simulink model "Autopilot_harness"  (Simulink 8.0)
settings: Solver=ode23  StartTime=0.0  StopTime=25  MaxStep=1/40  RelTol=1e-2  AbsTol=1e-3
model workspace (MAT data in the model file):
  tmp20121902TempDataBlockParam15378051 = 1
  tmp20121902TempDataBlockParam16564336 = 1
  tmp20121902TempDataBlockParam11960188 = 1
  beaver_init_roll = 0
  tmp2399823TempDataBlockParam8793363 = 1
  tmp2399823TempDataBlockParam27430435 = 11
  tmp2399823TempDataBlockParam30328219 : num (value not decoded)
PreLoadFcn:
  | Plant_data
values from neighbouring files (symbols this model uses):
  beaver_init_roll = 0    [Plant_data.m]
undefined symbols (not defined in the file or in its folder): sigbuilder_block
libraries: simulink x4, aerolibconvert2 x1, Plant x1
Description:
  | Fly the DeHavilland Beaver
  | 
  | This demonstration uses a pilot's joystick to allow you to fly the DeHavilland
  | Beaver modeled with Simulnk, and Aerospace Blockset.  This model has been
  | color coded to aid in locating Aerospace Blockset blocks. The red blocks are
  | Aerospace Blockset blocks, the orange blocks are subsystems containing
  | additional Aerospace Blockset blocks and the white blocks are Simulink blocks.
  | 
  | The DeHavilland Beaver model includes the airframe dynamics, including
  | aerodynamics. Effects of the environment are also modeled, such as wind profiles
  | for the landing phase. Visualization for this model is done via an interface to
  | FlightGear, a open source flight simulator package.
  | 
  | The DeHavilland Beaver was first flown in 1947. Today it is still prized by pilots
  | for its reliability and versatility. The DeHavilland Beaver can be operated on wheels,
  | skis or float landing gear.
  | 
  | Speed Max       110 kts
  | Altitude Max 10,000 ft
  | Range Max       400 nm
  | Load                     6 passengers
  | Crew                     1 member
  | 
  | For more information on the FlightGear interface, see the documentation.
settings Model: Creator=The MathWorks Inc.  LastModifiedBy=ssauvage  CovMetricSettings=dcmtrwe  CovHTMLOptions=-aTS=1 -bRG=1 -bTC=1 -hTR=0 -nFC=0 -scm=1 -bcm=1 -xEv=0  CovSaveSingleToWorkspaceVar=off  CovCumulativeReport=on  CovModelRefEnable=off  ExtModeTrigMode=oneshot  ExtModeArmWhenConnect=off  ExtModeAutoUpdateStatusClock=off
settings DataIOCC: LimitDataPoints=off  SignalLoggingSaveFormat=ModelDataLogs  SaveOutput=off  SaveTime=off  SignalLoggingName=tmp2399823SignalLoggingName
settings OptimizationCC: BlockReduction=off  ConditionallyExecuteInputs=off  InlineParams=on  UseIntDivNetSlope=on  InlineInvariantSignals=on  InitFltsAndDblsToZero=on  EfficientFloat2IntCast=on  OptimizeModelRefInitCode=on
settings DebuggingCC: SignalInfNanChecking=error  ReadBeforeWriteMsg=EnableAllAsError  WriteAfterWriteMsg=EnableAllAsError  WriteAfterReadMsg=EnableAllAsError  AlgebraicLoopMsg=error  ArtificialAlgebraicLoopMsg=error  SaveWithParameterizedLinksMsg=none  CheckExecutionContextPreStartOutputMsg=on  CheckExecutionContextRuntimeOutputMsg=on  BlockPriorityViolationMsg=error  MaxConsecutiveZCsMsg=warning  InheritedTsInSrcMsg=error  DiscreteInheritContinuousMsg=error  SigSpecEnsureSampleTimeMsg=error  CheckMatrixSingularityMsg=error  IntegerOverflowMsg=error  ParameterUnderflowMsg=error  ParameterPrecisionLossMsg=error  UnnecessaryDatatypeConvMsg=warning  VectorMatrixConversionMsg=warning  SignalLabelMismatchMsg=warning  UnconnectedInputMsg=error  UnconnectedOutputMsg=error  UnconnectedLineMsg=error  SFcnCompatibilityMsg=warning  BusObjectLabelMismatch=error  RootOutportRequireBusObject=error  AssertControl=DisableAll  ModelReferenceIOMsg=error  ModelReferenceIOMismatchMessage=error  UnknownTsInhSupMsg=error  ModelReferenceDataLoggingMessage=error
settings HardwareCC: ProdIntDivRoundTo=Zero  ProdEndianess=LittleEndian  ProdHWDeviceType=Generic->Custom  TargetHWDeviceType=32-bit Generic
settings ModelReferenceCC: CheckModelReferenceTargetMessage=none
settings RTWCC: SystemTargetFile=ert.tlc  TemplateMakefile=ert_default_tmf  Description=Real-Time Workshop Embedded Coder (no auto configuration)  RTWVerbose=off  ProcessScript=ert_make_rtw_hook  IncludeERTFirstTime=on
settings CodeAppCC: ForceParamTrailComments=on  IgnoreCustomStorageClasses=off  MangleLength=4  ReqsInCode=on
settings ERTTargetCC: TargetFcnLib=ansi_tfl_tmw.mat  CodeReplacementLibrary=ANSI_C  MultiwordLength=2048  GenerateSampleERTMain=on  IncludeMdlTerminateFcn=off  SuppressErrorStatus=on  SupportAbsoluteTime=off  SupportNonFinite=off  SupportComplex=off  InlinedParameterPlacement=NonHierarchical  ERTCustomFileTemplate=example_file_process.tlc  ConvertIfToSwitch=off  SuppressUnreachableDefaultCases=off

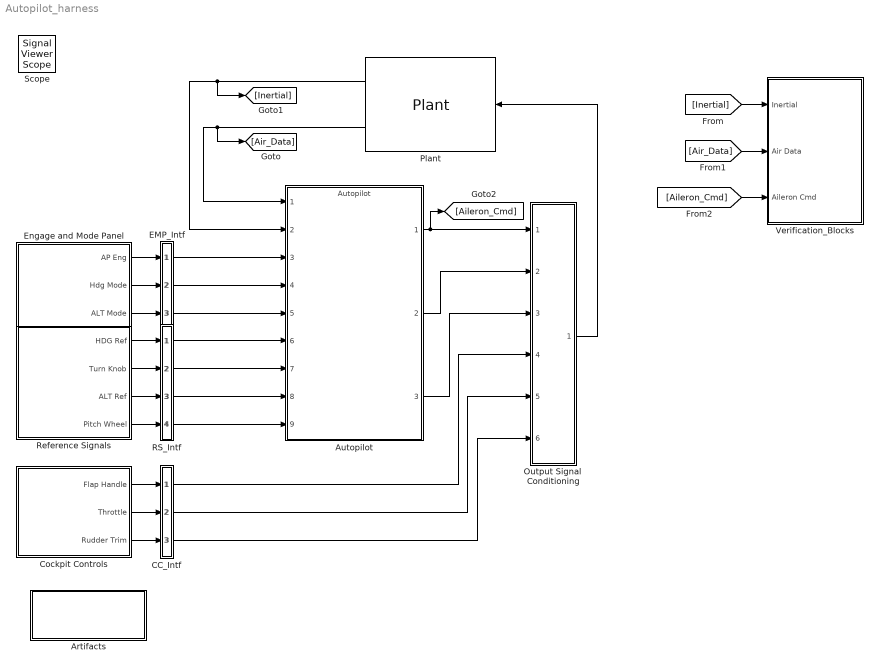
== system Autopilot_harness ==
  Artifacts : Subsystem
      mask Display: disp('View\nDO-178B Artifacts\n(double-click)');
  Autopilot : ModelReference  ModelNameDialog=Autopilot  SimulationMode=Normal  ModelReferenceVersion=1.155  CopyOfModelName=Autopilot  DefaultDataLogging=off
  CC_Intf : Subsystem
  Cockpit Controls : Subsystem  Tag=STV Subsys  LoadFcn=sigbuilder_block('load');  StartFcn=sigbuilder_block('start');  StopFcn=sigbuilder_block('stop');  ClipboardFcn=sigbuilder_block('clipboard');  mask(Sigbuilder block){}
      mask help: Sigbuilder GUI
      mask init:
      | if ~strcmp(get_param(bdroot(gcbh),'SimulationStatus'),'stopped') tuvar = sigbuilder_block('maskInit'); end
      settings: CopyFcn=sigbuilder_block('copy');  DeleteFcn=sigbuilder_block('delete');  ModelCloseFcn=sigbuilder_block('modelClose');  PreSaveFcn=sigbuilder_block('preSave');  PauseFcn=sigbuilder_block('pause')  ContinueFcn=sigbuilder_block('continue')  NameChangeFcn=sigbuilder_block('namechange');  OpenFcn=sigbuilder_block('open',[144.75 92.25 575.25 393 ]);  CloseFcn=sigbuilder_block('close');
      mask Display: plot(0,0,100,100,[10,10,40,40,10],[80,20,20,80,80],[40,10],[50,50], [40,27,10],[65,72,56],[40,25,25,10],[28,28,43,43]);
  EMP_Intf : Subsystem
  Engage and Mode Panel : Subsystem  Tag=STV Subsys  RequirementInfo={'other' 'do178b_autopilot_requirements.doc' '@1.2. Roll Hold Mode' 'true' '1.1. Roll Autopilot Engage Control' '' ; 'other' 'do178b_autopilot_requirements.doc' '1.2. Roll Hold Mode' 'true' '1.2. Roll Hold Mode' '' ; 'other' 'do178b_autopilot_requirements.doc' '1.1. Roll Autopilot Engage Control' 'true' '1.1. Roll Autopilot Engage Control' '' ; 'other' 'do178b_autopilot_requirements.doc' '1.8. Heading Hold Mode' 'true' '1.8. Heading Hold Mode' '' } %GIDa_8e9e9d99_d836_4084_a908_4b15c0f24bcd  LoadFcn=sigbuilder_block('load');  StartFcn=sigbuilder_block('start');  StopFcn=sigbuilder_block('stop');  ClipboardFcn=sigbuilder_block('clipboard');  mask(Sigbuilder block){}
      mask help: Sigbuilder GUI
      mask init:
      | if ~strcmp(get_param(bdroot(gcbh),'SimulationStatus'),'stopped') tuvar = sigbuilder_block('maskInit'); end
      settings: CopyFcn=sigbuilder_block('copy');  DeleteFcn=sigbuilder_block('delete');  ModelCloseFcn=sigbuilder_block('modelClose');  PreSaveFcn=sigbuilder_block('preSave');  PauseFcn=sigbuilder_block('pause')  ContinueFcn=sigbuilder_block('continue')  NameChangeFcn=sigbuilder_block('namechange');  OpenFcn=sigbuilder_block('open',[118.5 66 745.5 487.5 ]);  CloseFcn=sigbuilder_block('close');
      mask Display: plot(0,0,100,100,[10,10,40,40,10],[80,20,20,80,80],[40,10],[50,50], [40,27,10],[65,72,56],[40,25,25,10],[28,28,43,43]);
  Output Signal  Conditioning : Subsystem
  Plant : Plant/Plant  SystemSampleTime=-1
  RS_Intf : Subsystem
  Reference Signals : Subsystem  Tag=STV Subsys  RequirementInfo={'other' 'do178b_autopilot_requirements.doc' '1.3. Roll Hold Reference' 'true' '1.3. Roll Hold Reference' '' ; 'other' 'do178b_autopilot_requirements.doc' '1.9. Heading Hold Reference' 'true' '1.9. Heading Hold Reference' '' ; 'other' 'do178b_autopilot_requirements.doc' '1.3. Roll Hold Reference' 'true' '1.3. Roll Hold Reference' '' ; 'other' 'do178b_autopilot_requirements.doc' '1.3. Roll Hold Reference' 'true' '1.3. Roll Hold Reference' '' ; 'other' 'do178b_autopilot_requirements.doc' '1.3. Roll Hold Reference' 'true' '1.3. Roll Hold Reference' '' ; 'other' 'do178b_autopilot_requirements.doc' '1.3. Roll Hold Reference' 'true' '1.3. Roll Hold Reference' '' ; 'other' 'do178b_autopilot_requirements.doc' '1.3. Roll Hold Reference' 'true' '1.3. Roll Hold Reference' '' ; 'other' 'do178b_autopilot_requirements.doc' '1.3. Roll Hold Reference' 'true' '1.3. Roll Hold Reference' '' ; 'other' 'do178b_autopilot_requirements.doc' '1.4. Roll Performance' 'true' '1.4. Roll Performance' '' ; 'other' 'do178b_autopilot_requirements.doc' '1.4. Roll Performance' 'true' '1.4. Roll Performance' '' ; 'other' 'do178b_autopilot_requirements.doc' '1.4. Roll Performance' 'true' '1.4. Roll Performance' '' ; 'other' 'do178b_autopilot_requirements.doc' '1.5. Roll Rate Limit' 'true' '1.5. Roll Rate Limit' '' ; 'other' 'do178b_autopilot_requirements.doc' '1.6. Roll Angle Limit' 'true' '1.6. Roll Angle Limit' '' ; 'other' 'do178b_autopilot_requirements.doc' '1.4. Roll Performance' 'true' '1.4. Roll Performance' '' ; 'other' 'do178b_autopilot_requirements.doc' '1.5. Roll Rate Limit' 'true' '1.5. Roll Rate Limit' '' ; 'other' 'do178b_autopilot_requirements.doc' '1.6. Roll Angle Limit' 'true' '1.6. Roll Angle Limit' '' } %GIDa_9d9b9e1a_9cda_4488_bbc7_0b4cdaadb6f4  LoadFcn=sigbuilder_block('load');  StartFcn=sigbuilder_block('start');  StopFcn=sigbuilder_block('stop');  ClipboardFcn=sigbuilder_block('clipboard');  mask(Sigbuilder block){}
      mask help: Sigbuilder GUI
      mask init:
      | if ~strcmp(get_param(bdroot(gcbh),'SimulationStatus'),'stopped') tuvar = sigbuilder_block('maskInit'); end
      settings: CopyFcn=sigbuilder_block('copy');  DeleteFcn=sigbuilder_block('delete');  ModelCloseFcn=sigbuilder_block('modelClose');  PreSaveFcn=sigbuilder_block('preSave');  PauseFcn=sigbuilder_block('pause')  ContinueFcn=sigbuilder_block('continue')  NameChangeFcn=sigbuilder_block('namechange');  OpenFcn=sigbuilder_block('open',[124.5 -29.25 745.5 487.5 ]);  CloseFcn=sigbuilder_block('close');
      mask Display: plot(0,0,100,100,[10,10,40,40,10],[80,20,20,80,80],[40,10],[50,50], [40,27,10],[65,72,56],[40,25,25,10],[28,28,43,43]);
  Verification_Blocks : Subsystem
  Scope : SignalViewerScope  IOType=viewer  ZoomMode=yonly  RefreshTime=0.035000
  wires:
  Output Signal  Conditioning/1(Controls) -> Plant/1
  Autopilot/1 -> Output Signal  Conditioning/1(Aileron), [Aileron_Cmd]
  Plant/2 -> [Air_Data], Autopilot/1
  Plant/1 -> [Inertial], Autopilot/2
  Autopilot/2 -> Output Signal  Conditioning/2(Elevator)
  Autopilot/3 -> Output Signal  Conditioning/3(Rudder)
  Cockpit Controls/1(Flap Handle) -> CC_Intf/1(Flap Handle)
  Cockpit Controls/2(Throttle) -> CC_Intf/2("Throttle ")
  Engage and Mode Panel/1(AP Eng) -> EMP_Intf/1(AP Eng)
  Engage and Mode Panel/2(Hdg Mode) -> EMP_Intf/2(Hdg Mode)
  Engage and Mode Panel/3(ALT Mode) -> EMP_Intf/3(ALT Mode)
  Reference Signals/1(HDG Ref) -> RS_Intf/1(HDG Ref)
  Reference Signals/2(Turn Knob) -> RS_Intf/2(Turn Knob)
  Reference Signals/3(ALT Ref) -> RS_Intf/3(ALT Ref)
  Reference Signals/4(Pitch Wheel) -> RS_Intf/4(Pitch Wheel)
  EMP_Intf/1(AP_Eng) -> Autopilot/3
  EMP_Intf/2(Hdg_Mode) -> Autopilot/4
  EMP_Intf/3(ALT_Mode) -> Autopilot/5
  RS_Intf/1(HDG_Ref) -> Autopilot/6
  RS_Intf/2(Turn_Knob) -> Autopilot/7
  RS_Intf/3(ALT_Ref) -> Autopilot/8
  RS_Intf/4(Pitch_Wheel) -> Autopilot/9
  Cockpit Controls/3(Rudder Trim) -> CC_Intf/3(Rudder Trim)
  CC_Intf/1(Flap_Handle) -> Output Signal  Conditioning/4(Flap)
  CC_Intf/2(Throttle) -> Output Signal  Conditioning/5(Throttle)
  CC_Intf/3(Rudder_Trim) -> Output Signal  Conditioning/6(Rudder Trim)
  [Inertial] -> Verification_Blocks/1(Inertial)
  [Air_Data] -> Verification_Blocks/2(Air Data)
  [Aileron_Cmd] -> Verification_Blocks/3(Aileron Cmd)

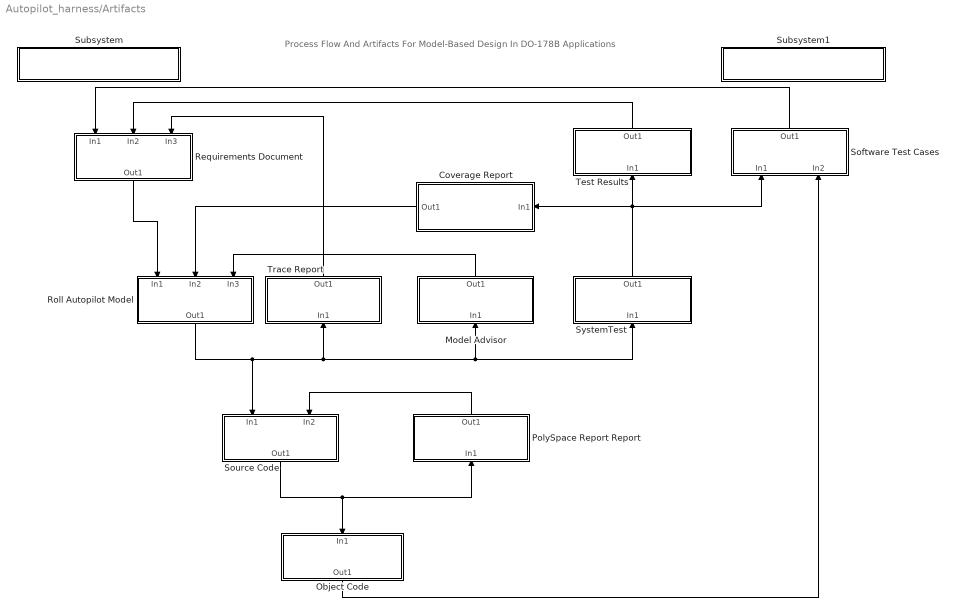
== system Autopilot_harness/Artifacts ==
  note: Process Flow And Artifacts For Model-Based Design In DO-178B Applications
  Coverage Report : Subsystem
      settings: OpenFcn=open('DO178B_Demo10203610.html');
      mask Display: disp('Open Model Coverage \nReport for Roll_AP \n (double-click)')
  Model Advisor : Subsystem
      settings: OpenFcn=|
      | open_system('roll_ap');
      | modeladvisor('roll_ap');
      mask Display: disp('Open Model Advisor \n for Roll_AP \n (double-click)')
  Object Code : Subsystem
      mask Display: disp('Compiled Object Code \n for Roll_AP')
  PolySpace Report Report : Subsystem
      settings: OpenFcn=winopen('results_roll_ap\misra_stats.csv');
      mask Display: disp('Polyspace Report \n for Roll_AP Code \n (double-click)')
  Requirements Document : Subsystem
      settings: OpenFcn=winopen('do178b_autopilot_requirements.doc');
      mask Display: disp('Open Requirements \n Document for Roll_AP \n (double-click)')
  Roll Autopilot Model : Subsystem
      settings: OpenFcn=open_system('roll_ap');
      mask Display: disp('Open Roll \n Autopilot Model \n (double-click)')
  Software Test Cases : Subsystem
      settings: OpenFcn=winopen('roll_ap_testcases(1).xls');
      mask Display: disp('Open Software Test \n Cases for Roll_AP \n (double-click)')
  Source Code : Subsystem
      settings: OpenFcn=open([pwd '\roll_ap_ert_rtw\html\roll_ap_codegen_rpt.html']);
      mask Display: disp('Open Code \n for Roll_AP \n (double-click)')
  Subsystem : Subsystem
      mask Display: disp('DO-178B Development Aritifacts');
  Subsystem1 : Subsystem
      mask Display: disp('DO-178B Verification Aritifacts');
  SystemTest : Subsystem
      settings: OpenFcn=systemtest('DO178B_Demo');
      mask Display: disp('Open SystemTest\n for DO178B_DHC2 \n (double-click)')
  Test Results : Subsystem
      settings: OpenFcn=|
      | %open('do178b_testreport.pdf');
      | open([pwd '\DO178B_Demo_report\DO178B_Demo_report.html']);
      mask Display: disp('Test Results Reports \n for DO178B_DHC2 \n (double-click)')
  Trace Report : Subsystem
      settings: OpenFcn=open('roll_ap_reqreport.html');
      mask Display: disp('Open Requirements \n Report for Roll_AP \n (double-click)')
  wires:
  PolySpace Report Report/1(Out1) -> Source Code/2(In2)
  Coverage Report/1(Out1) -> Roll Autopilot Model/2(In2)
  Object Code/1(Out1) -> Software Test Cases/2(In2)
  Software Test Cases/1(Out1) -> Requirements Document/1(In1)
  SystemTest/1(Out1) -> Software Test Cases/1(In1), Coverage Report/1(In1), Test Results/1(In1)
  Source Code/1(Out1) -> PolySpace Report Report/1(In1), Object Code/1(In1)
  Roll Autopilot Model/1(Out1) -> Source Code/1(In1), SystemTest/1(In1), Model Advisor/1(In1), Trace Report/1(In1)
  Test Results/1(Out1) -> Requirements Document/2(In2)
  Model Advisor/1(Out1) -> Roll Autopilot Model/3(In3)
  Trace Report/1(Out1) -> Requirements Document/3(In3)
  Requirements Document/1(Out1) -> Roll Autopilot Model/1(In1)

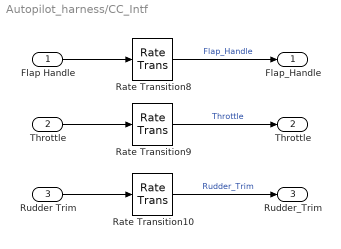
== system Autopilot_harness/CC_Intf ==
  Flap Handle : Inport
  "Throttle " : Inport  Port=2
  Rudder Trim : Inport  Port=3
  Rate Transition10 : RateTransition  OutPortSampleTime=1/40
  Rate Transition8 : RateTransition  OutPortSampleTime=1/40
  Rate Transition9 : RateTransition  OutPortSampleTime=1/40
  Flap_Handle : Outport
  Throttle : Outport  Port=2
  Rudder_Trim : Outport  Port=3
  wires:
  Flap Handle/1 -> Rate Transition8/1
  Rate Transition8/1 -> Flap_Handle/1  "Flap_Handle"
  "Throttle "/1 -> Rate Transition9/1
  Rate Transition9/1 -> Throttle/1  "Throttle"
  Rudder Trim/1 -> Rate Transition10/1
  Rate Transition10/1 -> Rudder_Trim/1  "Rudder_Trim"

== system Autopilot_harness/Cockpit Controls ==
  Demux : Demux  Tag=STV Demux  Outputs=3
  FromWs : FromWorkspace  Tag=STV FromWs  VariableName=tuvar  SampleTime=0  SigBuilderData=DataTag1  VnvData=DataTag2
      SigBuilderData=|
      | common.afterFinalStr = 'Extrapolate'
      | common.sampleTime = 0
      | dataSet.timeRange = [0 10]
      | dataSet.name = 'Steady State Flight'
      | sbobj.Groups.Name = 'Steady State Flight'
      | sbobj.Groups.Signals(1).Name = 'Flap Handle'
      | sbobj.Groups.Signals(1).XData = [0 10]
      | sbobj.Groups.Signals(1).YData = [0 0]
      | sbobj.Groups.Signals(2).Name = 'Throttle'
      | sbobj.Groups.Signals(2).XData = [0 10]
      | sbobj.Groups.Signals(2).YData = [0.625 0.625]
      | sbobj.Groups.Signals(3).Name = 'Rudder Trim'
      | sbobj.Groups.Signals(3).XData = [0 10]
      | sbobj.Groups.Signals(3).YData = [0 0]
  Flap Handle : Outport  Tag=STV Outport
  Throttle : Outport  Tag=STV Outport  Port=2
  Rudder Trim : Outport  Tag=STV Outport  Port=3
  wires:
  FromWs/1 -> Demux/1
  Demux/1 -> Flap Handle/1
  Demux/2 -> Throttle/1
  Demux/3 -> Rudder Trim/1

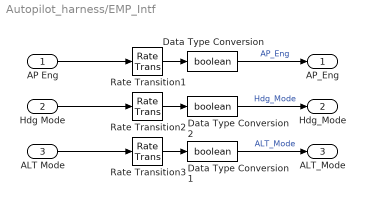
== system Autopilot_harness/EMP_Intf ==
  AP Eng : Inport
  Hdg Mode : Inport  Port=2
  ALT Mode : Inport  Port=3
  Data Type Conversion : DataTypeConversion  OutDataTypeStr=boolean
  Data Type Conversion1 : DataTypeConversion  OutDataTypeStr=boolean
  Data Type Conversion2 : DataTypeConversion  OutDataTypeStr=boolean
  Rate Transition1 : RateTransition  OutPortSampleTime=1/40
  Rate Transition2 : RateTransition  OutPortSampleTime=1/40
  Rate Transition3 : RateTransition  OutPortSampleTime=1/40
  AP_Eng : Outport
  Hdg_Mode : Outport  Port=2
  ALT_Mode : Outport  Port=3
  wires:
  AP Eng/1 -> Rate Transition1/1
  Data Type Conversion/1 -> AP_Eng/1  "AP_Eng"
  Hdg Mode/1 -> Rate Transition2/1
  Rate Transition2/1 -> Data Type Conversion2/1
  ALT Mode/1 -> Rate Transition3/1
  Rate Transition3/1 -> Data Type Conversion1/1
  Rate Transition1/1 -> Data Type Conversion/1
  Data Type Conversion2/1 -> Hdg_Mode/1  "Hdg_Mode"
  Data Type Conversion1/1 -> ALT_Mode/1  "ALT_Mode"

== system Autopilot_harness/Engage and Mode Panel ==
  Demux : Demux  Tag=STV Demux  Outputs=3
  FromWs : FromWorkspace  Tag=STV FromWs  VariableName=tuvar  SampleTime=0  SigBuilderData=DataTag3  VnvData=DataTag4
      SigBuilderData=|
      | common.afterFinalStr = 'Extrapolate'
      | common.sampleTime = 0
      | dataSet(1).timeRange = [0 25]
      | dataSet(1).name = 'Roll Hold Engage'
      | dataSet(2).timeRange = [0 25]
      | dataSet(2).name = 'Heading Hold Engage'
      | sbobj.Groups(1).Name = 'Roll Hold Engage'
      | sbobj.Groups(1).Signals(1).Name = 'AP Eng'
      | sbobj.Groups(1).Signals(1).XData = [0 0.1 0.1 25]
      | sbobj.Groups(1).Signals(1).YData = [0 0 1 1]
      | sbobj.Groups(1).Signals(2).Name = 'Hdg Mode'
      | sbobj.Groups(1).Signals(2).XData = [0 25]
      | sbobj.Groups(1).Signals(2).YData = [0 0]
      | sbobj.Groups(1).Signals(3).Name = 'ALT Mode'
      | sbobj.Groups(1).Signals(3).XData = [0 1 1 25]
      | sbobj.Groups(1).Signals(3).YData = [0 0 1 1]
      | sbobj.Groups(2).Name = 'Heading Hold Engage'
      | sbobj.Groups(2).Signals(1).Name = 'AP Eng'
      | sbobj.Groups(2).Signals(1).XData = [0 0.1 0.1 25]
      | sbobj.Groups(2).Signals(1).YData = [0 0 1 1]
      | sbobj.Groups(2).Signals(2).Name = 'Hdg Mode'
      | sbobj.Groups(2).Signals(2).XData = [0 1 1 25]
      | sbobj.Groups(2).Signals(2).YData = [0 0 1 1]
      | sbobj.Groups(2).Signals(3).Name = 'ALT Mode'
      | sbobj.Groups(2).Signals(3).XData = [0 1 1 25]
      | sbobj.Groups(2).Signals(3).YData = [0 0 1 1]
  AP Eng : Outport  Tag=STV Outport
  Hdg Mode : Outport  Tag=STV Outport  Port=2
  ALT Mode : Outport  Tag=STV Outport  Port=3
  wires:
  Demux/1 -> AP Eng/1
  FromWs/1 -> Demux/1
  Demux/2 -> Hdg Mode/1
  Demux/3 -> ALT Mode/1

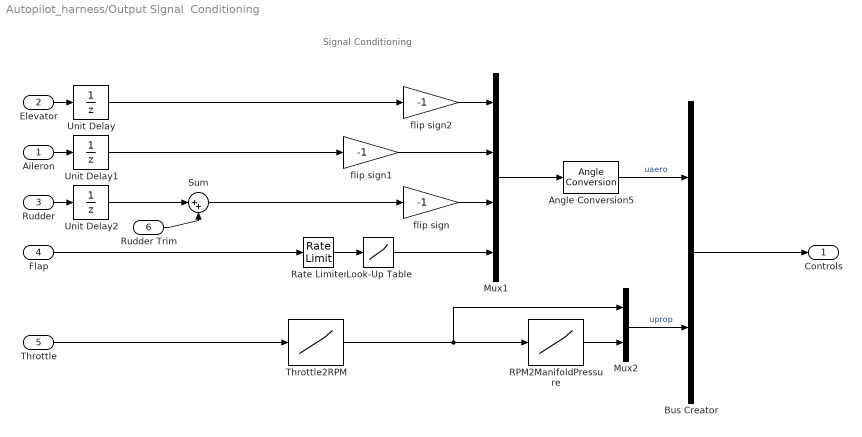
== system Autopilot_harness/Output Signal  Conditioning ==
  note: Signal Conditioning
  Aileron : Inport
  Elevator : Inport  Port=2
  Rudder : Inport  Port=3
  Flap : Inport  Port=4
  Throttle : Inport  Port=5
  Rudder Trim : Inport  Port=6
  Angle Conversion5 : aerolibconvert2/Angle Conversion  IU=deg  OU=rad
  Bus Creator : BusCreator  Inputs=2
  Look-Up Table : Lookup  InputValues=[0:3]  Table=[0 4 10 20]  SaturateOnIntegerOverflow=on
  Mux1 : Mux
  Mux2 : Mux  Inputs=2
  RPM2ManifoldPressure : Lookup_n-D  NumberOfTableDimensions=1  BreakpointsForDimension1=[0 1800 2300]  IndexSearchMethod=Linear search  BeginIndexSearchUsingPreviousIndexResult=on  Table=[0 22.5735 26]  ExtrapMethod=Clip  InputSameDT=on
  Rate Limiter : RateLimiter  RisingSlewLimit=0.5  FallingSlewLimit=-0.5
  Sum : Sum  Inputs=|++
  Throttle2RPM : Lookup_n-D  NumberOfTableDimensions=1  BreakpointsForDimension1=(1/6)*(3+([-3:3]))  IndexSearchMethod=Linear search  BeginIndexSearchUsingPreviousIndexResult=on  Table=((1+tanh([-3:3]))/(1+tanh(2.65))-0.0025)*2300  ExtrapMethod=Clip  InputSameDT=on
  Unit Delay : UnitDelay  SampleTime=-1
  Unit Delay1 : UnitDelay  SampleTime=-1
  Unit Delay2 : UnitDelay  SampleTime=-1
  flip sign : Gain  Gain=-1  SaturateOnIntegerOverflow=on  OutDataTypeStr=Inherit: Same as input  ParamDataTypeStr=Inherit: Same as input
  flip sign1 : Gain  Gain=-1  SaturateOnIntegerOverflow=on  OutDataTypeStr=Inherit: Same as input  ParamDataTypeStr=Inherit: Same as input
  flip sign2 : Gain  Gain=-1  SaturateOnIntegerOverflow=on  OutDataTypeStr=Inherit: Same as input  ParamDataTypeStr=Inherit: Same as input
  Controls : Outport
  wires:
  Bus Creator/1 -> Controls/1
  flip sign2/1 -> Mux1/1
  flip sign1/1 -> Mux1/2
  Throttle2RPM/1 -> RPM2ManifoldPressure/1, Mux2/1
  flip sign/1 -> Mux1/3
  Mux2/1 -> Bus Creator/2  "uprop"
  RPM2ManifoldPressure/1 -> Mux2/2
  Angle Conversion5/1 -> Bus Creator/1  "uaero"
  Mux1/1 -> Angle Conversion5/1
  Elevator/1 -> Unit Delay/1
  Aileron/1 -> Unit Delay1/1
  Look-Up Table/1 -> Mux1/4
  Rate Limiter/1 -> Look-Up Table/1
  Flap/1 -> Rate Limiter/1
  Throttle/1 -> Throttle2RPM/1
  Sum/1 -> flip sign/1
  Rudder/1 -> Unit Delay2/1
  Rudder Trim/1 -> Sum/2
  Unit Delay/1 -> flip sign2/1
  Unit Delay1/1 -> flip sign1/1
  Unit Delay2/1 -> Sum/1

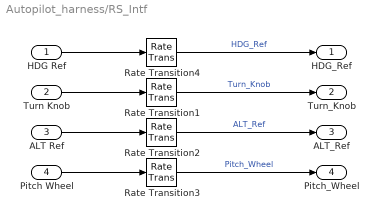
== system Autopilot_harness/RS_Intf ==
  HDG Ref : Inport
  Turn Knob : Inport  Port=2
  ALT Ref : Inport  Port=3
  Pitch Wheel : Inport  Port=4
  Rate Transition{1..4} (4 alike) : RateTransition  OutPortSampleTime=1/40
  HDG_Ref : Outport
  Turn_Knob : Outport  Port=2
  ALT_Ref : Outport  Port=3
  Pitch_Wheel : Outport  Port=4
  wires:
  HDG Ref/1 -> Rate Transition4/1
  Rate Transition4/1 -> HDG_Ref/1  "HDG_Ref"
  Turn Knob/1 -> Rate Transition1/1
  Rate Transition1/1 -> Turn_Knob/1  "Turn_Knob"
  ALT Ref/1 -> Rate Transition2/1
  Rate Transition2/1 -> ALT_Ref/1  "ALT_Ref"
  Pitch Wheel/1 -> Rate Transition3/1
  Rate Transition3/1 -> Pitch_Wheel/1  "Pitch_Wheel"

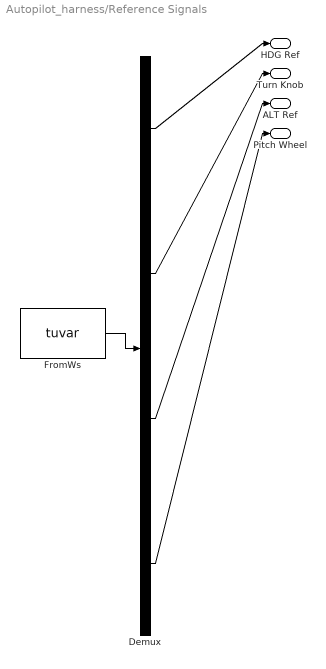
== system Autopilot_harness/Reference Signals ==
  Demux : Demux  Tag=STV Demux
  FromWs : FromWorkspace  Tag=STV FromWs  VariableName=tuvar  SampleTime=0  SigBuilderData=DataTag5  VnvData=DataTag6
      SigBuilderData=|
      | common.afterFinalStr = 'Extrapolate'
      | common.sampleTime = 0
      | dataSet(1).timeRange = [0 25]
      | dataSet(1).name = 'Trim Condition Engage'
      | dataSet(2).timeRange = [0 25]
      | dataSet(2).name = 'Turn Knob +2'
      | dataSet(3).timeRange = [0 25]
      | dataSet(3).name = 'Turn Knob -2'
      | dataSet(4).timeRange = [0 25]
      | dataSet(4).name = 'Turn Knob +4'
      | dataSet(5).timeRange = [0 25]
      | dataSet(5).name = 'Turn Knob -4'
      | dataSet(6).timeRange = [0 25]
      | dataSet(6).name = 'Turn Knob +30'
      | dataSet(7).timeRange = [0 25]
      | dataSet(7).name = 'Turn Knob -30'
      | dataSet(8).timeRange = [0 25]
      | dataSet(8).name = 'Roll Step - Positive'
      | dataSet(9).timeRange = [0 25]
      | dataSet(9).name = 'Roll Step - Negative'
      | dataSet(10).timeRange = [0 25]
      | dataSet(10).name = 'Roll Rate and Limit - Positive'
      | dataSet(11).timeRange = [0 25]
      | dataSet(11).name = 'Roll Rate and Limit - Negative'
      | sbobj.Groups(1).Name = 'Trim Condition Engage'
      | sbobj.Groups(1).Signals(1).Name = 'HDG Ref'
      | sbobj.Groups(1).Signals(1).XData = [0 25]
      | sbobj.Groups(1).Signals(1).YData = [113 113]
      | sbobj.Groups(1).Signals(2).Name = 'Turn Knob'
      | sbobj.Groups(1).Signals(2).XData = [0 25]
      | sbobj.Groups(1).Signals(2).YData = [0 0]
      | sbobj.Groups(1).Signals(3).Name = 'ALT Ref'
      | sbobj.Groups(1).Signals(3).XData = [0 25]
      | sbobj.Groups(1).Signals(3).YData = [7225 7225]
      | sbobj.Groups(1).Signals(4).Name = 'Pitch Wheel'
      | sbobj.Groups(1).Signals(4).XData = [0 25]
      | sbobj.Groups(1).Signals(4).YData = [0 0]
      | sbobj.Groups(2).Name = 'Turn Knob +2'
      | sbobj.Groups(2).Signals(1).Name = 'HDG Ref'
      | sbobj.Groups(2).Signals(1).XData = [0 25]
      | sbobj.Groups(2).Signals(1).YData = [113 113]
      | sbobj.Groups(2).Signals(2).Name = 'Turn Knob'
      | sbobj.Groups(2).Signals(2).XData = [0 25]
      | sbobj.Groups(2).Signals(2).YData = [2 2]
      | sbobj.Groups(2).Signals(3).Name = 'ALT Ref'
      | sbobj.Groups(2).Signals(3).XData = [0 25]
      | sbobj.Groups(2).Signals(3).YData = [7225 7225]
      | sbobj.Groups(2).Signals(4).Name = 'Pitch Wheel'
      | sbobj.Groups(2).Signals(4).XData = [0 25]
      | sbobj.Groups(2).Signals(4).YData = [0 0]
      | sbobj.Groups(3).Name = 'Turn Knob -2'
      | sbobj.Groups(3).Signals(1).Name = 'HDG Ref'
      | sbobj.Groups(3).Signals(1).XData = [0 25]
      | sbobj.Groups(3).Signals(1).YData = [113 113]
      | sbobj.Groups(3).Signals(2).Name = 'Turn Knob'
      | sbobj.Groups(3).Signals(2).XData = [0 25]
      | sbobj.Groups(3).Signals(2).YData = [-2 -2]
      | sbobj.Groups(3).Signals(3).Name = 'ALT Ref'
      | sbobj.Groups(3).Signals(3).XData = [0 25]
      | sbobj.Groups(3).Signals(3).YData = [7225 7225]
      | sbobj.Groups(3).Signals(4).Name = 'Pitch Wheel'
      | sbobj.Groups(3).Signals(4).XData = [0 25]
      | sbobj.Groups(3).Signals(4).YData = [0 0]
      | sbobj.Groups(4).Name = 'Turn Knob +4'
      | sbobj.Groups(4).Signals(1).Name = 'HDG Ref'
      | sbobj.Groups(4).Signals(1).XData = [0 25]
      | sbobj.Groups(4).Signals(1).YData = [113 113]
      | sbobj.Groups(4).Signals(2).Name = 'Turn Knob'
      | sbobj.Groups(4).Signals(2).XData = [0 25]
      | sbobj.Groups(4).Signals(2).YData = [4 4]
      | sbobj.Groups(4).Signals(3).Name = 'ALT Ref'
      | sbobj.Groups(4).Signals(3).XData = [0 25]
      | sbobj.Groups(4).Signals(3).YData = [7225 7225]
      | sbobj.Groups(4).Signals(4).Name = 'Pitch Wheel'
      | sbobj.Groups(4).Signals(4).XData = [0 25]
      | sbobj.Groups(4).Signals(4).YData = [0 0]
      | sbobj.Groups(5).Name = 'Turn Knob -4'
      | sbobj.Groups(5).Signals(1).Name = 'HDG Ref'
      | sbobj.Groups(5).Signals(1).XData = [0 25]
      | sbobj.Groups(5).Signals(1).YData = [113 113]
      | sbobj.Groups(5).Signals(2).Name = 'Turn Knob'
      | sbobj.Groups(5).Signals(2).XData = [0 25]
      | sbobj.Groups(5).Signals(2).YData = [-4 -4]
      | sbobj.Groups(5).Signals(3).Name = 'ALT Ref'
      | sbobj.Groups(5).Signals(3).XData = [0 25]
      | sbobj.Groups(5).Signals(3).YData = [7225 7225]
      | sbobj.Groups(5).Signals(4).Name = 'Pitch Wheel'
      | sbobj.Groups(5).Signals(4).XData = [0 25]
      | sbobj.Groups(5).Signals(4).YData = [0 0]
      | sbobj.Groups(6).Name = 'Turn Knob +30'
      | sbobj.Groups(6).Signals(1).Name = 'HDG Ref'
      | sbobj.Groups(6).Signals(1).XData = [0 25]
      | sbobj.Groups(6).Signals(1).YData = [113 113]
      | sbobj.Groups(6).Signals(2).Name = 'Turn Knob'
      | sbobj.Groups(6).Signals(2).XData = [0 25]
      | sbobj.Groups(6).Signals(2).YData = [30 30]
      | sbobj.Groups(6).Signals(3).Name = 'ALT Ref'
      | sbobj.Groups(6).Signals(3).XData = [0 25]
      | sbobj.Groups(6).Signals(3).YData = [7225 7225]
      | sbobj.Groups(6).Signals(4).Name = 'Pitch Wheel'
      | sbobj.Groups(6).Signals(4).XData = [0 25]
      | sbobj.Groups(6).Signals(4).YData = [0 0]
      | sbobj.Groups(7).Name = 'Turn Knob -30'
      | sbobj.Groups(7).Signals(1).Name = 'HDG Ref'
      | sbobj.Groups(7).Signals(1).XData = [0 25]
      | sbobj.Groups(7).Signals(1).YData = [113 113]
      | sbobj.Groups(7).Signals(2).Name = 'Turn Knob'
      | sbobj.Groups(7).Signals(2).XData = [0 25]
      | sbobj.Groups(7).Signals(2).YData = [-30 -30]
      | sbobj.Groups(7).Signals(3).Name = 'ALT Ref'
      | sbobj.Groups(7).Signals(3).XData = [0 25]
      | sbobj.Groups(7).Signals(3).YData = [7225 7225]
      | sbobj.Groups(7).Signals(4).Name = 'Pitch Wheel'
      | sbobj.Groups(7).Signals(4).XData = [0 25]
      | sbobj.Groups(7).Signals(4).YData = [0 0]
      | sbobj.Groups(8).Name = 'Roll Step - Positive'
      | sbobj.Groups(8).Signals(1).Name = 'HDG Ref'
      | sbobj.Groups(8).Signals(1).XData = [0 25]
      | sbobj.Groups(8).Signals(1).YData = [113 113]
      | sbobj.Groups(8).Signals(2).Name = 'Turn Knob'
      | sbobj.Groups(8).Signals(2).XData = [0 10 10 25]
      | sbobj.Groups(8).Signals(2).YData = [0 0 3 3]
      | sbobj.Groups(8).Signals(3).Name = 'ALT Ref'
      | sbobj.Groups(8).Signals(3).XData = [0 25]
      | sbobj.Groups(8).Signals(3).YData = [7225 7225]
      | sbobj.Groups(8).Signals(4).Name = 'Pitch Wheel'
      | sbobj.Groups(8).Signals(4).XData = [0 25]
      | sbobj.Groups(8).Signals(4).YData = [0 0]
      | sbobj.Groups(9).Name = 'Roll Step - Negative'
      | sbobj.Groups(9).Signals(1).Name = 'HDG Ref'
      | sbobj.Groups(9).Signals(1).XData = [0 25]
      | sbobj.Groups(9).Signals(1).YData = [113 113]
      | sbobj.Groups(9).Signals(2).Name = 'Turn Knob'
      | sbobj.Groups(9).Signals(2).XData = [0 10 10 25]
      | sbobj.Groups(9).Signals(2).YData = [0 0 -3 -3]
      | sbobj.Groups(9).Signals(3).Name = 'ALT Ref'
      | sbobj.Groups(9).Signals(3).XData = [0 25]
      | sbobj.Groups(9).Signals(3).YData = [7225 7225]
      | sbobj.Groups(9).Signals(4).Name = 'Pitch Wheel'
      | sbobj.Groups(9).Signals(4).XData = [0 25]
      | sbobj.Groups(9).Signals(4).YData = [0 0]
      | sbobj.Groups(10).Name = 'Roll Rate and Limit - Positive'
      | sbobj.Groups(10).Signals(1).Name = 'HDG Ref'
      | sbobj.Groups(10).Signals(1).XData = [0 25]
      | sbobj.Groups(10).Signals(1).YData = [113 113]
      | sbobj.Groups(10).Signals(2).Name = 'Turn Knob'
      | sbobj.Groups(10).Signals(2).XData = [0 10 10 25]
      | sbobj.Groups(10).Signals(2).YData = [0 0 35 35]
      | sbobj.Groups(10).Signals(3).Name = 'ALT Ref'
      | sbobj.Groups(10).Signals(3).XData = [0 25]
      | sbobj.Groups(10).Signals(3).YData = [7225 7225]
      | sbobj.Groups(10).Signals(4).Name = 'Pitch Wheel'
      | sbobj.Groups(10).Signals(4).XData = [0 25]
      | sbobj.Groups(10).Signals(4).YData = [0 0]
      | sbobj.Groups(11).Name = 'Roll Rate and Limit - Negative'
      | sbobj.Groups(11).Signals(1).Name = 'HDG Ref'
      | sbobj.Groups(11).Signals(1).XData = [0 25]
      | sbobj.Groups(11).Signals(1).YData = [113 113]
      | sbobj.Groups(11).Signals(2).Name = 'Turn Knob'
      | sbobj.Groups(11).Signals(2).XData = [0 10 10 25]
      | sbobj.Groups(11).Signals(2).YData = [0 0 -35 -35]
      | sbobj.Groups(11).Signals(3).Name = 'ALT Ref'
      | sbobj.Groups(11).Signals(3).XData = [0 25]
      | sbobj.Groups(11).Signals(3).YData = [7225 7225]
      | sbobj.Groups(11).Signals(4).Name = 'Pitch Wheel'
      | sbobj.Groups(11).Signals(4).XData = [0 25]
      | sbobj.Groups(11).Signals(4).YData = [0 0]
  HDG Ref : Outport  Tag=STV Outport
  Turn Knob : Outport  Tag=STV Outport  Port=2
  ALT Ref : Outport  Tag=STV Outport  Port=3
  Pitch Wheel : Outport  Tag=STV Outport  Port=4
  wires:
  FromWs/1 -> Demux/1
  Demux/1 -> HDG Ref/1
  Demux/2 -> Turn Knob/1
  Demux/3 -> ALT Ref/1
  Demux/4 -> Pitch Wheel/1

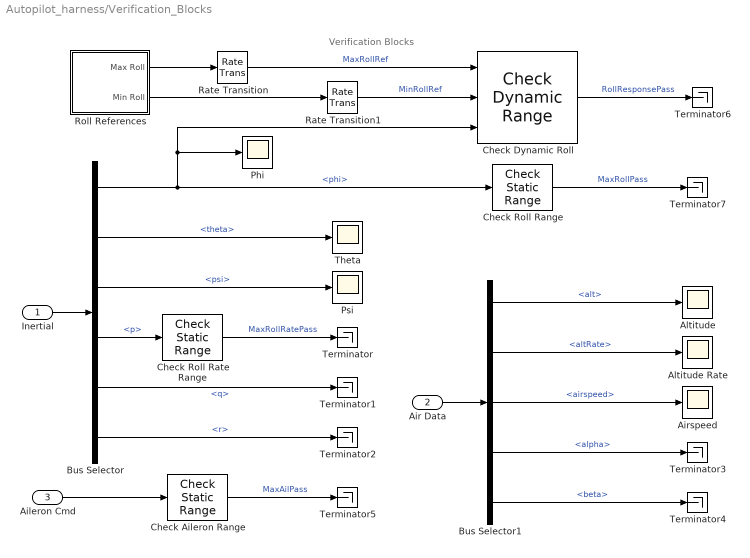
== system Autopilot_harness/Verification_Blocks ==
  note: Verification Blocks
  Inertial : Inport
  Air Data : Inport  Port=2
  Aileron Cmd : Inport  Port=3
  Airspeed : Scope
      settings: SaveName=ScopeData5
  Altitude : Scope
      settings: SaveName=ScopeData3
  Altitude Rate : Scope
      settings: SaveName=ScopeData4
  Bus Selector : BusSelector  OutputSignals=phi,theta,psi,p,q,r
  Bus Selector1 : BusSelector  OutputSignals=alt,altRate,airspeed,alpha,beta
  Check Aileron Range : simulink/Model Verification/Check  Static Range  Description=-15 <= u <= 15  max=15  max_included=on  min=-15  min_included=on  enabled=on  stopWhenAssertionFail=off  export=on  icon=graphic
      settings: AttributesFormatString=%<Description>
  Check Dynamic Roll : simulink/Model Verification/Check  Dynamic Range  Description=min < sig < max  enabled=on  stopWhenAssertionFail=off  export=on  icon=graphic
  Check Roll Range : simulink/Model Verification/Check  Static Range  Description=-33 <= u <= 33  max=33  max_included=on  min=-33  min_included=on  enabled=on  stopWhenAssertionFail=off  export=on  icon=graphic
      settings: AttributesFormatString=%<Description>
  Check Roll Rate Range : simulink/Model Verification/Check  Static Range  Description=-6.6 <= u <= 6.6  max=6.6  max_included=on  min=-6.6  min_included=on  enabled=on  stopWhenAssertionFail=off  export=on  icon=graphic
      settings: AttributesFormatString=%<Description>
  Phi : Scope
      settings: YMin=-32  YMax=-28
  Psi : Scope
      settings: SaveName=ScopeData2
  Rate Transition : RateTransition  X0=beaver_init_roll/pi*180+1  OutPortSampleTime=1/40
  Rate Transition1 : RateTransition  X0=beaver_init_roll/pi*180-1  OutPortSampleTime=1/40
  Roll References : Subsystem  Tag=STV Subsys  RequirementInfo={'other' 'do178b_autopilot_requirements.doc' '1.1. Roll Autopilot Engage Control' 'true' '1.1. Roll Autopilot Engage Control' '' ; 'other' 'do178b_autopilot_requirements.doc' '@1.2. Roll Hold Mode' 'true' '1.2. Roll Hold Mode' ' ' ; 'other' 'do178b_autopilot_requirements.doc' '@1.3. Roll Hold Reference' 'true' '1.3. Roll Hold Reference' ' ' ; 'other' 'do178b_autopilot_requirements.doc' '1.1. Roll Autopilot Engage Control' 'true' '1.1. Roll Autopilot Engage Control' '' ; 'other' 'do178b_autopilot_requirements.doc' '1.2. Roll Hold Mode' 'true' '1.2. Roll Hold Mode' '' ; 'other' 'do178b_autopilot_requirements.doc' '1.3. Roll Hold Reference' 'true' '1.3. Roll Hold Reference' '' ; 'other' 'do178b_autopilot_requirements.doc' '1.1. Roll Autopilot Engage Control' 'true' '1.1. Roll Autopilot Engage Control' '' ; 'other' 'do178b_autopilot_requirements.doc' '1.2. Roll Hold Mode' 'true' '1.2. Roll Hold Mode' '' ; 'other' 'do178b_autopilot_requirements.doc' '1.3. Roll Hold Reference' 'true' '1.3. Roll Hold Reference' '' ; 'other' 'do178b_autopilot_requirements.doc' '1.1. Roll Autopilot Engage Control' 'true' '1.1. Roll Autopilot Engage Control' '' ; 'other' 'do178b_autopilot_requirements.doc' '1.2. Roll Hold Mode' 'true' '1.2. Roll Hold Mode' '' ; 'other' 'do178b_autopilot_requirements.doc' '1.3. Roll Hold Reference' 'true' '1.3. Roll Hold Reference' '' ; 'other' 'do178b_autopilot_requirements.doc' '1.1. Roll Autopilot Engage Control' 'true' '1.1. Roll Autopilot Engage Control' '' ; 'other' 'do178b_autopilot_requirements.doc' '1.2. Roll Hold Mode' 'true' '1.2. Roll Hold Mode' '' ; 'other' 'do178b_autopilot_requirements.doc' '1.3. Roll Hold Reference' 'true' '1.3. Roll Hold Reference' '' ; 'other' 'do178b_autopilot_requirements.doc' '1.1. Roll Autopilot Engage Control' 'true' '1.1. Roll Autopilot Engage Control' '' ; 'other' 'do178b_autopilot_requirements.doc' '1.2. Roll Hold Mode' 'true' '1.2. Roll Hold Mode' '' ; 'other' 'do178b_autopilot_requirements.doc' '1.3. Roll Hold Reference' 'true' '1.3. Roll Hold Reference' '' ; 'other' 'do178b_autopilot_requirements.doc' '1.1. Roll Autopilot Engage Control' 'true' '1.1. Roll Autopilot Engage Control' '' ; 'other' 'do178b_autopilot_requirements.doc' '1.2. Roll Hold Mode' 'true' '1.2. Roll Hold Mode' '' ; 'other' 'do178b_autopilot_requirements.doc' '1.3. Roll Hold Reference' 'true' '1.3. Roll Hold Reference' '' ; 'other' 'do178b_autopilot_requirements.doc' '1.1. Roll Autopilot Engage Control' 'true' '1.1. Roll Autopilot Engage Control' '' ; 'other' 'do178b_autopilot_requirements.doc' '1.2. Roll Hold Mode' 'true' '1.2. Roll Hold Mode' '' ; 'other' 'do178b_autopilot_requirements.doc' '1.3. Roll Hold Reference' 'true' '1.3. Roll Hold Reference' '' ; 'other' 'do178b_autopilot_requirements.doc' '1.1. Roll Autopilot Engage Control' 'true' '1.1. Roll Autopilot Engage Control' '' ; 'other' 'do178b_autopilot_requirements.doc' '1.2. Roll Hold Mode' 'true' '1.2. Roll Hold Mode' '' ; 'other' 'do178b_autopilot_requirements.doc' '1.3. Roll Hold Reference' 'true' '1.3. Roll Hold Reference' '' ; 'other' 'do178b_autopilot_requirements.doc' '1.1. Roll Autopilot Engage Control' 'true' '1.1. Roll Autopilot Engage Control' '' ; 'other' 'do178b_autopilot_requirements.doc' '1.2. Roll Hold Mode' 'true' '1.2. Roll Hold Mode' '' ; 'other' 'do178b_autopilot_requirements.doc' '1.3. Roll Hold Reference' 'true' '1.3. Roll Hold Reference' '' ; 'other' 'do178b_autopilot_requirements.doc' '1.1. Roll Autopilot Engage Control' 'true' '1.1. Roll Autopilot Engage Control' '' ; 'other' 'do178b_autopilot_requirements.doc' '1.2. Roll Hold Mode' 'true' '1.2. Roll Hold Mode' '' ; 'other' 'do178b_autopilot_requirements.doc' '1.3. Roll Hold Reference' 'true' '1.3. Roll Hold Reference' '' ; 'other' 'do178b_autopilot_requirements.doc' '1.1. Roll Autopilot Engage Control' 'true' '1.1. Roll Autopilot Engage Control' '' ; 'other' 'do178b_autopilot_requirements.doc' '1.2. Roll Hold Mode' 'true' '1.2. Roll Hold Mode' '' ; 'other' 'do178b_autopilot_requirements.doc' '1.3. Roll Hold Reference' 'true' '1.3. Roll Hold Reference' '' ; 'other' 'do178b_autopilot_requirements.doc' '1.1. Roll Autopilot Engage Control' 'true' '1.1. Roll Autopilot Engage Control' '' ; 'other' 'do178b_autopilot_requirements.doc' '1.2. Roll Hold Mode' 'true' '1.2. Roll Hold Mode' '' ; 'other' 'do178b_autopilot_requirements.doc' '1.3. Roll Hold Reference' 'true' '1.3. Roll Hold Reference' '' ; 'other' 'do178b_autopilot_requirements.doc' '1.1. Roll Autopilot Engage Control' 'true' '1.1. Roll Autopilot Engage Control' '' ; 'other' 'do178b_autopilot_requirements.doc' '1.2. Roll Hold Mode' 'true' '1.2. Roll Hold Mode' '' ; 'other' 'do178b_autopilot_requirements.doc' '1.3. Roll Hold Reference' 'true' '1.3. Roll Hold Reference' '' ; 'other' 'do178b_autopilot_requirements.doc' '1.1. Roll Autopilot Engage Control' 'true' '1.1. Roll Autopilot Engage Control' '' ; 'other' 'do178b_autopilot_requirements.doc' '1.2. Roll Hold Mode' 'true' '1.2. Roll Hold Mode' '' ; 'other' 'do178b_autopilot_requirements.doc' '1.3. Roll Hold Reference' 'true' '1.3. Roll Hold Reference' '' ; 'other' 'do178b_autopilot_requirements.doc' '1.1. Roll Autopilot Engage Control' 'true' '1.1. Roll Autopilot Engage Control' '' ; 'other' 'do178b_autopilot_requirements.doc' '1.2. Roll Hold Mode' 'true' '1.2. Roll Hold Mode' '' ; 'other' 'do178b_autopilot_requirements.doc' '1.3. Roll Hold Reference' 'true' '1.3. Roll Hold Reference' '' ; 'other' 'do178b_autopilot_requirements.doc' '1.4. Roll Performance' 'true' '1.4. Roll Performance' '' ; 'other' 'do178b_autopilot_requirements.doc' '1.4. Roll Performance' 'true' '1.4. Roll Performance' '' ; 'other' 'do178b_autopilot_requirements.doc' '1.5. Roll Rate Limit' 'true' '1.5. Roll Rate Limit' '' ; 'other' 'do178b_autopilot_requirements.doc' '1.6. Roll Angle Limit' 'true' '1.6. Roll Angle Limit' '' ; 'other' 'do178b_autopilot_requirements.doc' '1.7. Aileron Angle Limit' 'true' '1.7. Aileron Angle Limit' '' ; 'other' 'do178b_autopilot_requirements.doc' '@1.5. Roll Rate Limit' 'true' '1.5. Roll Rate Limit' ' ' ; 'other' 'do178b_autopilot_requirements.doc' '@1.6. Roll Angle Limit' 'true' '1.6. Roll Angle Limit' ' ' ; 'other' 'do178b_autopilot_requirements.doc' '1.7. Aileron Angle Limit' 'true' '1.7. Aileron Angle Limit' '' } %GIDa_ba1e5288_f274_4b44_a12a_943497d6d101  LoadFcn=sigbuilder_block('load');  StartFcn=sigbuilder_block('start');  StopFcn=sigbuilder_block('stop');  ClipboardFcn=sigbuilder_block('clipboard');  mask(Sigbuilder block){}
      mask help: Sigbuilder GUI
      mask init:
      | if ~strcmp(get_param(bdroot(gcbh),'SimulationStatus'),'stopped') tuvar = sigbuilder_block('maskInit'); end
      settings: CopyFcn=sigbuilder_block('copy');  DeleteFcn=sigbuilder_block('delete');  ModelCloseFcn=sigbuilder_block('modelClose');  PreSaveFcn=sigbuilder_block('preSave');  PauseFcn=sigbuilder_block('pause')  ContinueFcn=sigbuilder_block('continue')  NameChangeFcn=sigbuilder_block('namechange');  OpenFcn=sigbuilder_block('open',[18.75 136.5 707.25 385.5 ]);  CloseFcn=sigbuilder_block('close');
      mask Display: plot(0,0,100,100,[10,10,40,40,10],[80,20,20,80,80],[40,10],[50,50], [40,27,10],[65,72,56],[40,25,25,10],[28,28,43,43]);
  Terminator{,1..7} (8 alike) : Terminator
  Theta : Scope
  wires:
  Inertial/1 -> Bus Selector/1
  Air Data/1 -> Bus Selector1/1
  Bus Selector/1 -> Check Roll Range/1, Check Dynamic Roll/3, Phi/1  "<phi>"
  Bus Selector/2 -> Theta/1  "<theta>"
  Bus Selector/3 -> Psi/1  "<psi>"
  Bus Selector/4 -> Check Roll Rate Range/1  "<p>"
  Bus Selector/5 -> Terminator1/1  "<q>"
  Bus Selector/6 -> Terminator2/1  "<r>"
  Bus Selector1/1 -> Altitude/1  "<alt>"
  Bus Selector1/2 -> Altitude Rate/1  "<altRate>"
  Bus Selector1/3 -> Airspeed/1  "<airspeed>"
  Bus Selector1/4 -> Terminator3/1  "<alpha>"
  Bus Selector1/5 -> Terminator4/1  "<beta>"
  Aileron Cmd/1 -> Check Aileron Range/1
  Check Aileron Range/1 -> Terminator5/1  "MaxAilPass"
  Check Roll Rate Range/1 -> Terminator/1  "MaxRollRatePass"
  Check Dynamic Roll/1 -> Terminator6/1  "RollResponsePass"
  Roll References/1(Max Roll) -> Rate Transition/1
  Roll References/2(Min Roll) -> Rate Transition1/1
  Check Roll Range/1 -> Terminator7/1  "MaxRollPass"
  Rate Transition/1 -> Check Dynamic Roll/1  "MaxRollRef"
  Rate Transition1/1 -> Check Dynamic Roll/2  "MinRollRef"

== system Autopilot_harness/Artifacts/Coverage Report ==
  In1 : Inport
  Ground : Ground
  Terminator : Terminator
  Out1 : Outport
  wires:
  In1/1 -> Terminator/1
  Ground/1 -> Out1/1

== system Autopilot_harness/Artifacts/Model Advisor ==
  In1 : Inport
  Ground : Ground
  Terminator : Terminator
  Out1 : Outport
  wires:
  In1/1 -> Terminator/1
  Ground/1 -> Out1/1

== system Autopilot_harness/Artifacts/Object Code ==
  In1 : Inport
  Ground : Ground
  Terminator : Terminator
  Out1 : Outport
  wires:
  Ground/1 -> Out1/1
  In1/1 -> Terminator/1

== system Autopilot_harness/Artifacts/PolySpace Report Report ==
  In1 : Inport
  Ground : Ground
  Terminator : Terminator
  Out1 : Outport
  wires:
  Ground/1 -> Out1/1
  In1/1 -> Terminator/1

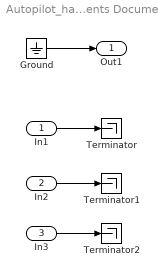
== system Autopilot_harness/Artifacts/Requirements Document ==
  In1 : Inport
  In2 : Inport  Port=2
  In3 : Inport  Port=3
  Ground : Ground
  Terminator : Terminator
  Terminator1 : Terminator
  Terminator2 : Terminator
  Out1 : Outport
  wires:
  In3/1 -> Terminator2/1
  In2/1 -> Terminator1/1
  In1/1 -> Terminator/1
  Ground/1 -> Out1/1

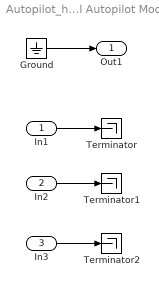
== system Autopilot_harness/Artifacts/Roll Autopilot Model ==
  In1 : Inport
  In2 : Inport  Port=2
  In3 : Inport  Port=3
  Ground : Ground
  Terminator : Terminator
  Terminator1 : Terminator
  Terminator2 : Terminator
  Out1 : Outport
  wires:
  In2/1 -> Terminator1/1
  In1/1 -> Terminator/1
  Ground/1 -> Out1/1
  In3/1 -> Terminator2/1

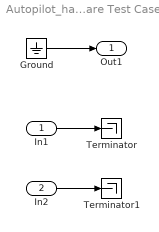
== system Autopilot_harness/Artifacts/Software Test Cases ==
  In1 : Inport
  In2 : Inport  Port=2
  Ground : Ground
  Terminator : Terminator
  Terminator1 : Terminator
  Out1 : Outport
  wires:
  In2/1 -> Terminator1/1
  In1/1 -> Terminator/1
  Ground/1 -> Out1/1

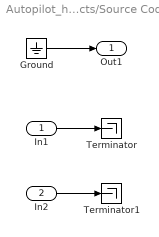
== system Autopilot_harness/Artifacts/Source Code ==
  In1 : Inport
  In2 : Inport  Port=2
  Ground : Ground
  Terminator : Terminator
  Terminator1 : Terminator
  Out1 : Outport
  wires:
  In2/1 -> Terminator1/1
  In1/1 -> Terminator/1
  Ground/1 -> Out1/1

== system Autopilot_harness/Artifacts/Subsystem ==

== system Autopilot_harness/Artifacts/Subsystem1 ==

== system Autopilot_harness/Artifacts/SystemTest ==
  In1 : Inport
  Ground : Ground
  Terminator : Terminator
  Out1 : Outport
  wires:
  In1/1 -> Terminator/1
  Ground/1 -> Out1/1

== system Autopilot_harness/Artifacts/Test Results ==
  In1 : Inport
  Ground : Ground
  Terminator : Terminator
  Out1 : Outport
  wires:
  Ground/1 -> Out1/1
  In1/1 -> Terminator/1

== system Autopilot_harness/Artifacts/Trace Report ==
  In1 : Inport
  Ground : Ground
  Terminator : Terminator
  Out1 : Outport
  wires:
  In1/1 -> Terminator/1
  Ground/1 -> Out1/1

== system Autopilot_harness/Verification_Blocks/Roll References ==
  Demux : Demux  Tag=STV Demux  Outputs=2
  FromWs : FromWorkspace  Tag=STV FromWs  VariableName=tuvar  SampleTime=0  SigBuilderData=DataTag7  VnvData=DataTag8
      SigBuilderData=|
      | common.afterFinalStr = 'Extrapolate'
      | common.sampleTime = 0
      | dataSet(1).timeRange = [0 25]
      | dataSet(1).name = 'Roll Test 1'
      | dataSet(2).timeRange = [0 25]
      | dataSet(2).name = 'Roll Test 2'
      | dataSet(3).timeRange = [0 25]
      | dataSet(3).name = 'Roll Test 3'
      | dataSet(4).timeRange = [0 25]
      | dataSet(4).name = 'Roll Test 4'
      | dataSet(5).timeRange = [0 25]
      | dataSet(5).name = 'Roll Test 5'
      | dataSet(6).timeRange = [0 25]
      | dataSet(6).name = 'Roll Test 6'
      | dataSet(7).timeRange = [0 25]
      | dataSet(7).name = 'Roll Test 7'
      | dataSet(8).timeRange = [0 25]
      | dataSet(8).name = 'Roll Test 8'
      | dataSet(9).timeRange = [0 25]
      | dataSet(9).name = 'Roll Test 9'
      | dataSet(10).timeRange = [0 25]
      | dataSet(10).name = 'Roll Test 10'
      | dataSet(11).timeRange = [0 25]
      | dataSet(11).name = 'Roll Test 11'
      | dataSet(12).timeRange = [0 25]
      | dataSet(12).name = 'Roll Test 12'
      | dataSet(13).timeRange = [0 25]
      | dataSet(13).name = 'Roll Test 13'
      | dataSet(14).timeRange = [0 25]
      | dataSet(14).name = 'Roll Test 14'
      | dataSet(15).timeRange = [0 25]
      | dataSet(15).name = 'Roll Test 15'
      | dataSet(16).timeRange = [0 25]
      | dataSet(16).name = 'Roll Test 16'
      | dataSet(17).timeRange = [0 25]
      | dataSet(17).name = 'Roll Test 17'
      | dataSet(18).timeRange = [0 25]
      | dataSet(18).name = 'Roll Test 18'
      | dataSet(19).timeRange = [0 25]
      | dataSet(19).name = 'Roll Test 19'
      | dataSet(20).timeRange = [0 25]
      | dataSet(20).name = 'Roll Test 20'
      | sbobj.Groups(1).Name = 'Roll Test 1'
      | sbobj.Groups(1).Signals(1).Name = 'Max Roll'
      | sbobj.Groups(1).Signals(1).XData = [0 25]
      | sbobj.Groups(1).Signals(1).YData = [1 1]
      | sbobj.Groups(1).Signals(2).Name = 'Min Roll'
      | sbobj.Groups(1).Signals(2).XData = [0 25]
      | sbobj.Groups(1).Signals(2).YData = [-1 -1]
      | sbobj.Groups(2).Name = 'Roll Test 2'
      | sbobj.Groups(2).Signals(1).Name = 'Max Roll'
      | sbobj.Groups(2).Signals(1).XData = [0 2.1 2.1 6.1 6.1 25]
      | sbobj.Groups(2).Signals(1).YData = [4.1 4.1 1.6 1.6 1 1]
      | sbobj.Groups(2).Signals(2).Name = 'Min Roll'
      | sbobj.Groups(2).Signals(2).XData = [0 25]
      | sbobj.Groups(2).Signals(2).YData = [-1 -1]
      | sbobj.Groups(3).Name = 'Roll Test 3'
      | sbobj.Groups(3).Signals(1).Name = 'Max Roll'
      | sbobj.Groups(3).Signals(1).XData = [0 25]
      | sbobj.Groups(3).Signals(1).YData = [1 1]
      | sbobj.Groups(3).Signals(2).Name = 'Min Roll'
      | sbobj.Groups(3).Signals(2).XData = [0 2.1 2.1 6.1 6.1 25]
      | sbobj.Groups(3).Signals(2).YData = [-4.1 -4.1 -1.6 -1.6 -1 -1]
      | sbobj.Groups(4).Name = 'Roll Test 4'
      | sbobj.Groups(4).Signals(1).Name = 'Max Roll'
      | sbobj.Groups(4).Signals(1).XData = [0 25]
      | sbobj.Groups(4).Signals(1).YData = [9 9]
      | sbobj.Groups(4).Signals(2).Name = 'Min Roll'
      | sbobj.Groups(4).Signals(2).XData = [0 25]
      | sbobj.Groups(4).Signals(2).YData = [7 7]
      | sbobj.Groups(5).Name = 'Roll Test 5'
      | sbobj.Groups(5).Signals(1).Name = 'Max Roll'
      | sbobj.Groups(5).Signals(1).XData = [0 25]
      | sbobj.Groups(5).Signals(1).YData = [-7 -7]
      | sbobj.Groups(5).Signals(2).Name = 'Min Roll'
      | sbobj.Groups(5).Signals(2).XData = [0 25]
      | sbobj.Groups(5).Signals(2).YData = [-9 -9]
      | sbobj.Groups(6).Name = 'Roll Test 6'
      | sbobj.Groups(6).Signals(1).Name = 'Max Roll'
      | sbobj.Groups(6).Signals(1).XData = [0 25]
      | sbobj.Groups(6).Signals(1).YData = [29 29]
      | sbobj.Groups(6).Signals(2).Name = 'Min Roll'
      | sbobj.Groups(6).Signals(2).XData = [0 25]
      | sbobj.Groups(6).Signals(2).YData = [27 27]
      | sbobj.Groups(7).Name = 'Roll Test 7'
      | sbobj.Groups(7).Signals(1).Name = 'Max Roll'
      | sbobj.Groups(7).Signals(1).XData = [0 25]
      | sbobj.Groups(7).Signals(1).YData = [-27 -27]
      | sbobj.Groups(7).Signals(2).Name = 'Min Roll'
      | sbobj.Groups(7).Signals(2).XData = [0 25]
      | sbobj.Groups(7).Signals(2).YData = [-29 -29]
      | sbobj.Groups(8).Name = 'Roll Test 8'
      | sbobj.Groups(8).Signals(1).Name = 'Max Roll'
      | sbobj.Groups(8).Signals(1).XData = [0 6.1 6.1 25]
      | sbobj.Groups(8).Signals(1).YData = [32.1 32.1 31 31]
      | sbobj.Groups(8).Signals(2).Name = 'Min Roll'
      | sbobj.Groups(8).Signals(2).XData = [0 25]
      | sbobj.Groups(8).Signals(2).YData = [29 29]
      | sbobj.Groups(9).Name = 'Roll Test 9'
      | sbobj.Groups(9).Signals(1).Name = 'Max Roll'
      | sbobj.Groups(9).Signals(1).XData = [0 25]
      | sbobj.Groups(9).Signals(1).YData = [-29 -29]
      | sbobj.Groups(9).Signals(2).Name = 'Min Roll'
      | sbobj.Groups(9).Signals(2).XData = [0 6.1 6.1 25]
      | sbobj.Groups(9).Signals(2).YData = [-32.1 -32.1 -31 -31]
      | sbobj.Groups(10).Name = 'Roll Test 10'
      | sbobj.Groups(10).Signals(1).Name = 'Max Roll'
      | sbobj.Groups(10).Signals(1).XData = [0 25]
      | sbobj.Groups(10).Signals(1).YData = [1 1]
      | sbobj.Groups(10).Signals(2).Name = 'Min Roll'
      | sbobj.Groups(10).Signals(2).XData = [0 25]
      | sbobj.Groups(10).Signals(2).YData = [-1 -1]
      | sbobj.Groups(11).Name = 'Roll Test 11'
      | sbobj.Groups(11).Signals(1).Name = 'Max Roll'
      | sbobj.Groups(11).Signals(1).XData = [0 25]
      | sbobj.Groups(11).Signals(1).YData = [1 1]
      | sbobj.Groups(11).Signals(2).Name = 'Min Roll'
      | sbobj.Groups(11).Signals(2).XData = [0 25]
      | sbobj.Groups(11).Signals(2).YData = [-1 -1]
      | sbobj.Groups(12).Name = 'Roll Test 12'
      | sbobj.Groups(12).Signals(1).Name = 'Max Roll'
      | sbobj.Groups(12).Signals(1).XData = [0 25]
      | sbobj.Groups(12).Signals(1).YData = [1 1]
      | sbobj.Groups(12).Signals(2).Name = 'Min Roll'
      | sbobj.Groups(12).Signals(2).XData = [0 25]
      | sbobj.Groups(12).Signals(2).YData = [-1 -1]
      | sbobj.Groups(13).Name = 'Roll Test 13'
      | sbobj.Groups(13).Signals(1).Name = 'Max Roll'
      | sbobj.Groups(13).Signals(1).XData = [0 0.1 0.6 4 4 25]
      | sbobj.Groups(13).Signals(1).YData = [0.95 1 5 5.05 5 5]
      | sbobj.Groups(13).Signals(2).Name = 'Min Roll'
      | sbobj.Groups(13).Signals(2).XData = [0 6.1 6.1 25]
      | sbobj.Groups(13).Signals(2).YData = [-1 -1 3 3]
      | sbobj.Groups(14).Name = 'Roll Test 14'
      | sbobj.Groups(14).Signals(1).Name = 'Max Roll'
      | sbobj.Groups(14).Signals(1).XData = [0 6.1 6.1 25]
      | sbobj.Groups(14).Signals(1).YData = [1 1 -3 -3]
      | sbobj.Groups(14).Signals(2).Name = 'Min Roll'
      | sbobj.Groups(14).Signals(2).XData = [0 0.1 0.6 25]
      | sbobj.Groups(14).Signals(2).YData = [-1 -1 -5 -5]
      | sbobj.Groups(15).Name = 'Roll Test 15'
      | sbobj.Groups(15).Signals(1).Name = 'Max Roll'
      | sbobj.Groups(15).Signals(1).XData = [0 0.1 4.5 25]
      | sbobj.Groups(15).Signals(1).YData = [1 1 31 31]
      | sbobj.Groups(15).Signals(2).Name = 'Min Roll'
      | sbobj.Groups(15).Signals(2).XData = [0 2.1 9.6 25]
      | sbobj.Groups(15).Signals(2).YData = [-1 -1 29 29]
      | sbobj.Groups(16).Name = 'Roll Test 16'
      | sbobj.Groups(16).Signals(1).Name = 'Max Roll'
      | sbobj.Groups(16).Signals(1).XData = [0 2.1 9.6 25]
      | sbobj.Groups(16).Signals(1).YData = [1 1 -29 -29]
      | sbobj.Groups(16).Signals(2).Name = 'Min Roll'
      | sbobj.Groups(16).Signals(2).XData = [0 0.1 0.6 4.5 25]
      | sbobj.Groups(16).Signals(2).YData = [-1 -1 -4 -31 -31]
      | sbobj.Groups(17).Name = 'Roll Test 17'
      | sbobj.Groups(17).Signals(1).Name = 'Max Roll'
      | sbobj.Groups(17).Signals(1).XData = [0 10 10 25]
      | sbobj.Groups(17).Signals(1).YData = [1 1 4 4]
      | sbobj.Groups(17).Signals(2).Name = 'Min Roll'
      | sbobj.Groups(17).Signals(2).XData = [0 12 12 14 14 25]
      | sbobj.Groups(17).Signals(2).YData = [-1 -1 1.6 1.6 2 2]
      | sbobj.Groups(18).Name = 'Roll Test 18'
      | sbobj.Groups(18).Signals(1).Name = 'Max Roll'
      | sbobj.Groups(18).Signals(1).XData = [0 12 12 14 14 25]
      | sbobj.Groups(18).Signals(1).YData = [1 1 -1.6 -1.6 -2 -2]
      | sbobj.Groups(18).Signals(2).Name = 'Min Roll'
      | sbobj.Groups(18).Signals(2).XData = [0 10 10 25]
      | sbobj.Groups(18).Signals(2).YData = [-1 -1 -4 -4]
      | sbobj.Groups(19).Name = 'Roll Test 19'
      | sbobj.Groups(19).Signals(1).Name = 'Max Roll'
      | sbobj.Groups(19).Signals(1).XData = [0 10 15 25]
      | sbobj.Groups(19).Signals(1).YData = [1 1 33 33]
      | sbobj.Groups(19).Signals(2).Name = 'Min Roll'
      | sbobj.Groups(19).Signals(2).XData = [0 12 19 25]
      | sbobj.Groups(19).Signals(2).YData = [-1 -1 29 29]
      | sbobj.Groups(20).Name = 'Roll Test 20'
      | sbobj.Groups(20).Signals(1).Name = 'Max Roll'
      | sbobj.Groups(20).Signals(1).XData = [0 12 19 25]
      | sbobj.Groups(20).Signals(1).YData = [1 1 -29 -29]
      | sbobj.Groups(20).Signals(2).Name = 'Min Roll'
      | sbobj.Groups(20).Signals(2).XData = [0 10 15 25]
      | sbobj.Groups(20).Signals(2).YData = [-1 -1 -33 -33]
  Max Roll : Outport  Tag=STV Outport
  Min Roll : Outport  Tag=STV Outport  Port=2
  wires:
  Demux/1 -> Max Roll/1
  FromWs/1 -> Demux/1
  Demux/2 -> Min Roll/1
